simulink model "photovoltaic_single_phase_gridconnected_inverter_5kW"  (R2020b)
settings: Solver=FixedStepDiscrete  StartTime=0.0  StopTime=6  FixedStep=5e-7  MaxStep=1e-6  RelTol=1e-3
undefined symbols (not defined in the file): DiscIntNeverNeededParam, sigbuilder_block
libraries: powerlib x20, pid_lib x2, discretizing x2, re_lib x1, powerlib_meascontrol x1
settings Model: SimulationMode=accelerator  Creator=zhaoy  LastModifiedBy=Administrator
settings DataIOCC: ReturnWorkspaceOutputs=off
settings OptimizationCC: LifeSpan=inf
settings DebuggingCC: ArithmeticOperatorsInVariantConditions=warning
settings SFSimCC: SimUseLocalCustomCode=off  CustomCodeUndefinedFunction=UseInterfaceOnly
settings RTWCC: RTWUseLocalCustomCode=off
settings CodeAppCC: StateflowObjectComments=on
settings SimscapeCC: SimscapeNormalizeSystem=off

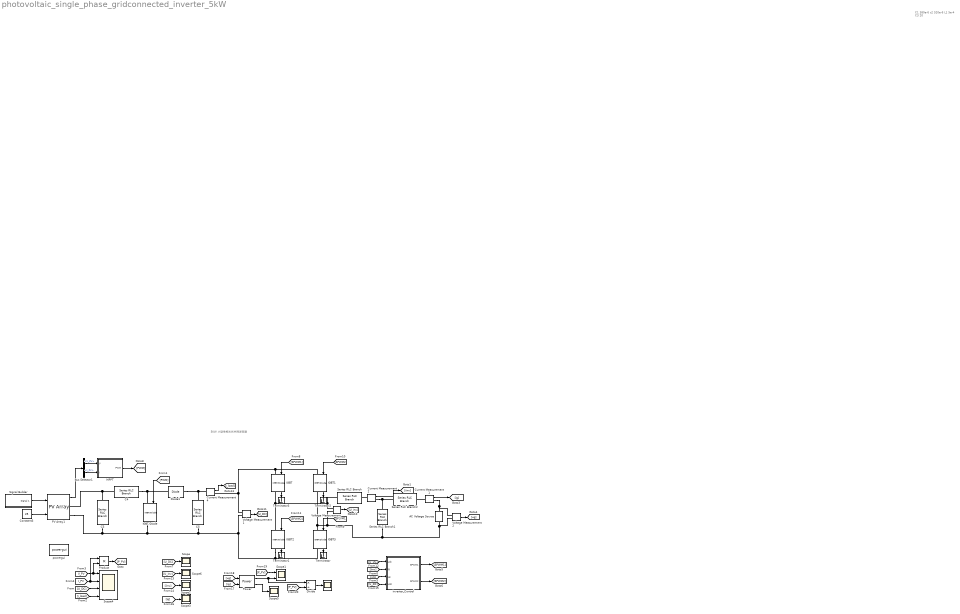
== system photovoltaic_single_phase_gridconnected_inverter_5kW ==
  note: 5KW 小型单相光伏并网逆变器
  note: C1 380e-6
      | c2 520e-6
      | L1 5e-4
      | C3 20
  " " : Scope
  AC Voltage Source : powerlib/Electrical Sources/AC Voltage Source  Amplitude=311  Phase=0  Frequency=50  SampleTime=0  Measurements=None  BusType=swing  Pref=10e3  Qref=0  Qmin=-inf  Qmax=+inf
  Bus Selector1 : BusSelector  OutputSignals=V_PV,I_PV
  C3 : powerlib/Elements/Series RLC Branch  LConnTagsString=__new0  RConnTagsString=__new0  BranchType=C  Resistance=1e-4  Inductance=3.05e-3  SetiL0=off  InitialCurrent=0  Capacitance=500e-6  Setx0=off  InitialVoltage=0  Measurements=Branch voltage
  C4 : powerlib/Elements/Series RLC Branch  LConnTagsString=__new0  RConnTagsString=__new0  BranchType=RL  Resistance=0.01  Inductance=2e-3  SetiL0=off  InitialCurrent=0  Capacitance=100e-6  Setx0=off  InitialVoltage=0  Measurements=Branch voltage
  C5 : powerlib/Elements/Series RLC Branch  LConnTagsString=__new0  RConnTagsString=__new0  BranchType=C  Resistance=1e-4  Inductance=3.05e-3  SetiL0=off  InitialCurrent=0  Capacitance=3000e-6  Setx0=off  InitialVoltage=0  Measurements=Branch voltage
  Constant3 : Constant  Value=25
  Current Measurement1 : powerlib/Measurements/Current Measurement  PhasorSimulation=off  OutputType=Complex  PSBequivalent=0
  Current Measurement2 : powerlib/Measurements/Current Measurement  PhasorSimulation=off  OutputType=Complex  PSBequivalent=0
  Current Measurement4 : powerlib/Measurements/Current Measurement  PhasorSimulation=off  OutputType=Complex  PSBequivalent=0
  Diode1 : powerlib/Power Electronics/Diode  Ron=0.001  Lon=0  Vf=0.8  IC=0  UseSnubber=off  Rs=500  Cs=250e-9  Measurements=off
  Divide : Product  Inputs=*/
  IGBT{,1..3} (4 alike) : powerlib/Power Electronics/IGBT//Diode  Ron=1e-3  Rs=1e5  Cs=inf  Measurements=on
  IGBT/Diode : powerlib/Power Electronics/IGBT//Diode  Ron=1e-3  Rs=1e5  Cs=inf  Measurements=on
  MPPT : Subsystem
  PV Array1 : re_lib/Solar/PV Array  Npar=3  Nser=8  PlotType=array @ 25 deg.C & specified irradiances  S_vec=[600 1000 800]  Temp_C_vec="[ 45 25  ]"  ModuleName=User-defined  PlotWhenSelected=off  Pm=213.15  Ncell=60  Voc=36.3  Isc=7.84  Vm=29  Im=7.35  beta_Voc_pc=-0.36099  alpha_Isc_pc=0.102  beta_Voc=-0.13104  alpha_Isc=0.0079968  IL=7.8654  I0=2.9273e-10  nI=0.98119  Rsh=313.0553  Rs=0.39381  RobustModel=off  RobustCellTemperature=313.3991  BAL=on  Tc=1e-6  Tfilter=5e-5
  Power : powerlib_meascontrol/Measurements/Power  Freq=50  Vinit=[1, 0]  Iinit=[1, 0]  Ts=1e-6
  Product : Product
  Scope{,2..3,5..6} (5 alike) : Scope
  Scope1 : Scope  NumInputPorts=2
  Scope4 : Scope  NumInputPorts=4
  Series RLC Branch : powerlib/Elements/Series RLC Branch  LConnTagsString=__new0  RConnTagsString=__new0  BranchType=L  Resistance=0.01  Inductance=4.06e-3  SetiL0=off  InitialCurrent=0  Capacitance=1e-6  Setx0=off  InitialVoltage=0  Measurements=None
  Series RLC Branch1 : powerlib/Elements/Series RLC Branch  LConnTagsString=__new0  RConnTagsString=__new0  BranchType=C  Resistance=0.01  Inductance=20e-3  SetiL0=off  InitialCurrent=0  Capacitance=6.23e-6  Setx0=off  InitialVoltage=0  Measurements=None
  Series RLC Branch2 : powerlib/Elements/Series RLC Branch  LConnTagsString=__new0  RConnTagsString=__new0  BranchType=L  Resistance=0.01  Inductance=4.35e-3  SetiL0=off  InitialCurrent=0  Capacitance=1e-6  Setx0=off  InitialVoltage=0  Measurements=None
  Signal Builder : Subsystem  Tag=STV Subsys  LoadFcn=sigbuilder_block('load');  StartFcn=sigbuilder_block('start');  StopFcn=sigbuilder_block('stop');  ClipboardFcn=sigbuilder_block('clipboard');  mask(Sigbuilder block){tuvar=[0:10]}
      mask help: Simulink:masks:SigbuilderBlock_MD
      mask init:
      | if ~strcmp(get_param(bdroot(gcbh),'SimulationStatus'),'stopped') tuvar = sigbuilder_block('maskInit'); end
      settings: CopyFcn=sigbuilder_block('copy');  DeleteFcn=sigbuilder_block('delete');  ModelCloseFcn=sigbuilder_block('modelClose');  PreSaveFcn=sigbuilder_block('preSave');  PauseFcn=sigbuilder_block('pause');  ContinueFcn=sigbuilder_block('continue');  NameChangeFcn=sigbuilder_block('namechange');  OpenFcn=sigbuilder_block('open',[437.6 199.2 550.4 400 ]);  CloseFcn=sigbuilder_block('close');
      mask Display: plot(0, 0, 100, 100,[2, 2, 32, 32, 2], [68, 8, 8, 68, 68],[32, 2], [38, 38], [32, 19, 2],[53, 60, 44], [32, 17, 17, 2],[16, 16, 31, 31]);txt = getActiveGroup(gcbh);text(2, 100, txt,'verticalAlignment', 'top');
  Terminator{,1..3} (4 alike) : Terminator
  Voltage Measurement1 : powerlib/Measurements/Voltage Measurement  PhasorSimulation=off  OutputType=Complex  PSBequivalent=0
  Voltage Measurement2 : powerlib/Measurements/Voltage Measurement  PhasorSimulation=off  OutputType=Complex  PSBequivalent=0
  Voltage Measurement3 : powerlib/Measurements/Voltage Measurement  PhasorSimulation=off  OutputType=Complex  PSBequivalent=0
  inverter_Control : Subsystem
  powergui : powerlib/powergui  Priority=1  SimulationMode=Discrete  SampleTime=1e-6  frequency=50  Iterations=50  frequencyindice=50  Pbase=100e6  ErrMax=1e-4  UnitsV=kV  UnitsW=MW  buscounter=0  FunctionMessages=off  echomessages=off  EnableUseOfTLC=off  CurrentSourceSwitches=off  DisableSnubberDevices=off  DisableRonSwitches=off  DisableVfSwitches=off  DisplayEquations=off  AutomaticDiscreteSolvers=off  SolverType=Tustin/Backward Euler (TBE)  Interpol=off  ExternalGateDelay=off  methode=off  Ts=10  x0status=blocks  SPID=off  SwTol=0  HookPort=off  NonlinearTolerance=1e-4  nMaxIteration=100  ContinueOnMaxIteration=off  RestoreLinks=warning  ResistiveCurrentMeasurement=off  Frange=[0:2:500]  Ylog=off  Xlog=on  ShowGrid=off  save=off  variable=ZData  structure=ScopeData2  ZoomFFT=off  StartTime=1  cycles=40  DisplayStyle=2  fundamental=50  FreqAxis=on  MaxFrequency=1000  frequencyindicesteady=1  RmsSteady=2  display=off
  wires:
  Constant3/1 -> PV Array1/2
  Signal Builder/1(Signal 1) -> PV Array1/1
  PV Array1/1 -> Bus Selector1/1
  Voltage Measurement1/1 -> [U_DC]
  Current Measurement4/1 -> [i_load]
  [U_DC] -> Scope4/3
  [i_load] -> Scope4/4
  [V_PV] -> Product/2, Scope4/1
  [I_PV] -> Product/1, Scope4/2
  Current Measurement1/1 -> [ig]
  [SPWM1] -> IGBT/1
  [SPWM2] -> IGBT1/1
  Voltage Measurement2/1 -> [ug]
  [SPWM1] -> IGBT3/1
  [SPWM2] -> IGBT2/1
  inverter_Control/2(SPWM2) -> [SPWM2]
  [U_DC] -> inverter_Control/1(udc)
  [iinv] -> inverter_Control/2(Ig)
  inverter_Control/1(SPWM1) -> [SPWM1]
  Current Measurement2/1 -> [iinv]
  [ug] -> inverter_Control/3(ug)
  [U_DC] -> inverter_Control/4(Udc)
  Voltage Measurement3/1 -> [U_inv]
  [PWM] -> IGBT/Diode/1
  Bus Selector1/1 -> MPPT/1(V)  "<V_PV>"
  Bus Selector1/2 -> MPPT/2(I)  "<I_PV>"
  IGBT3/1 -> Terminator/1
  IGBT2/1 -> Terminator1/1
  IGBT1/1 -> Terminator2/1
  IGBT/1 -> Terminator3/1
  MPPT/1(PWM) -> [PWM]
  [U_DC] -> Scope/1
  [U_inv] -> Scope6/1
  [iinv] -> Scope2/1
  [ig] -> Scope3/1
  Product/1 -> [P_PV]
  [ig] -> Power/2
  [ug] -> Power/1
  Power/2 -> Scope5/1
  [P_PV] -> Scope1/1
  Power/1 -> Divide/1, Scope1/2
  Divide/1 -> " "/1
  [P_PV] -> Divide/2
  connections:
  IGBT3/RConn1 -- PV Array1/RConn2 -- C3/RConn1 -- IGBT/Diode/RConn1 -- C5/RConn1 -- Voltage Measurement1/LConn2 -- IGBT2/RConn1
  Current Measurement4/LConn1 -- Diode1/RConn1 -- C5/LConn1
  IGBT/LConn1 -- Voltage Measurement1/LConn1 -- Current Measurement4/RConn1 -- IGBT1/LConn1
  Voltage Measurement2/LConn1 -- Current Measurement1/RConn1 -- AC Voltage Source/RConn1
  Voltage Measurement2/LConn2 -- Series RLC Branch1/RConn1 -- Voltage Measurement3/LConn2 -- IGBT1/RConn1 -- IGBT3/LConn1 -- AC Voltage Source/LConn1
  Series RLC Branch/LConn1 -- Voltage Measurement3/LConn1 -- IGBT/RConn1 -- IGBT2/LConn1
  Current Measurement2/LConn1 -- Series RLC Branch/RConn1
  Current Measurement2/RConn1 -- Series RLC Branch2/LConn1 -- Series RLC Branch1/LConn1
  Current Measurement1/LConn1 -- Series RLC Branch2/RConn1
  C3/LConn1 -- C4/LConn1 -- PV Array1/RConn1
  C4/RConn1 -- Diode1/LConn1 -- IGBT/Diode/LConn1

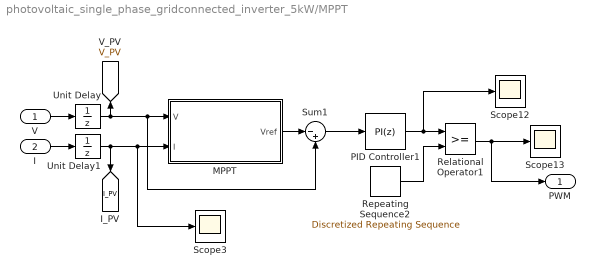
== system photovoltaic_single_phase_gridconnected_inverter_5kW/MPPT ==
  V : Inport
  I : Inport  Port=2
  MPPT : MATLAB Function  TreatAsAtomicUnit=on
  PID Controller1 : pid_lib/PID Controller  Controller=PI  Form=Parallel  TimeDomain=Discrete-time  UseExternalTs=off  SampleTime=-1  IntegratorMethod=Forward Euler  FilterMethod=Forward Euler  ControllerParametersSource=internal  P=0.005  I=0.0075  D=0  UseFilter=on  N=100  TunerSelectOption=Transfer Function Based (PID Tuner App)  InitialConditionSource=internal  InitialConditionForIntegrator=0  InitialConditionForFilter=0  DifferentiatorICPrevScaledInput=0  ExternalReset=none  TrackingMode=off  Kt=1  LimitOutput=off  SatLimitsSource=internal  UpperSaturationLimit=inf  LowerSaturationLimit=-inf  LinearizeAsGain=on  AntiWindupMode=none  Kb=1  POutMin=[]  POutMax=[]  IOutMin=[]  IOutMax=[]  DOutMin=[]  DOutMax=[]  NOutMin=[]  NOutMax=[]  SumOutMin=[]  SumOutMax=[]  SaturationOutMin=[]  SaturationOutMax=[]  PParamMin=[]  PParamMax=[]  IParamMin=[]  IParamMax=[]  DParamMin=[]  DParamMax=[]  NParamMin=[]  NParamMax=[]  KbParamMin=[]  KbParamMax=[]  KtParamMin=[]  KtParamMax=[]  KbOutMin=[]  KbOutMax=[]  KtOutMin=[]  KtOutMax=[]  IntegratorOutMin=[]  IntegratorOutMax=[]  FilterOutMin=[]  FilterOutMax=[]  SumI1OutMin=[]  SumI1OutMax=[]  SumI2OutMin=[]  SumI2OutMax=[]  SumI3OutMin=[]  SumI3OutMax=[]  SumI4OutMin=[]  SumI4OutMax=[]  SumDOutMin=[]  SumDOutMax=[]  DifferentiatorOutMin=[]  DifferentiatorOutMax=[]  FilterDiffOutCoefMin=[]  FilterDiffOutCoefMax=[]  ReciprocalOutMin=[]  ReciprocalOutMax=[]  SumDenOutMin=[]  SumDenOutMax=[]  SumNumOutMin=[]  SumNumOutMax=[]  DivideOutMin=[]  DivideOutMax=[]  UdiffTsProdOutMin=[]  UdiffTsProdOutMax=[]  NTsProdOutMin=[]  NTsProdOutMax=[]  UintegralTsProdOutMin=[]  UintegralTsProdOutMax=[]  UngainTsProdOutMin=[]  UngainTsProdOutMax=[]  IntegratorContinuousStateAttributes=''  IntegratorStateMustResolveToSignalObject=off  IntegratorRTWStateStorageClass=Auto  FilterContinuousStateAttributes=''  FilterStateMustResolveToSignalObject=off  FilterRTWStateStorageClass=Auto  ParallelPVariant=InternalParameters  IdealPVariant=Disabled  IVariant=InternalParameters  DVariant=Disabled  IntegratorVariant=Discrete  SatVariant=Disabled  AWVariant=Passthrough  PCopyVariant=Disabled  TRVariant=Disabled  FdbkBlocksVariant=Forward  IdealPFdbkVariant=Disabled  SatFdbkVariant=Disabled  DerivativeFilterVariant=Disabled  NVariant=Disabled  NCopyVariant=Disabled_SignalSpec  FilterICVariant=Disabled  IntegratorICVariant=InternalICs  ExternalResetVariant=Disabled  TRSumVariant=Passthrough  SumFdbkVariant=Disabled  SumVariant=Sum_PI  TsampFilterVariant=InternalTs  TsampNgainVariant=Passthrough  TsampIntegralVariant=Passthrough  ExternalSaturationOutDataTypeStr=Inherit: Same as second input
  Relational Operator1 : RelationalOperator  OutDataTypeStr=boolean  RndMeth=Simplest
  Repeating Sequence2 : discretizing/Discretized Repeating Sequence  rep_seq_t=[0 0.0001 0.0002]  rep_seq_y=[0 1 0]  SampleTime=1e-6
      settings: SourceProductBaseCode=SL
  Scope12 : Scope
  Scope13 : Scope
  Scope3 : Scope
  Sum1 : Sum  Inputs=|-+
  Unit Delay : UnitDelay  SampleTime=1e-5  HasFrameUpgradeWarning=on
  Unit Delay1 : UnitDelay  SampleTime=1e-5  HasFrameUpgradeWarning=on
  PWM : Outport
  tag scope: I_PV=global, V_PV=global
  wires:
  Relational Operator1/1 -> PWM/1, Scope13/1
  Unit Delay1/1 -> [I_PV], MPPT/2(I), Scope3/1
  MPPT/1(Vref) -> Sum1/1
  PID Controller1/1 -> Scope12/1, Relational Operator1/1
  Repeating Sequence2/1 -> Relational Operator1/2
  Sum1/1 -> PID Controller1/1
  V/1 -> Unit Delay/1
  I/1 -> Unit Delay1/1
  Unit Delay/1 -> [V_PV], MPPT/1(V), Sum1/2

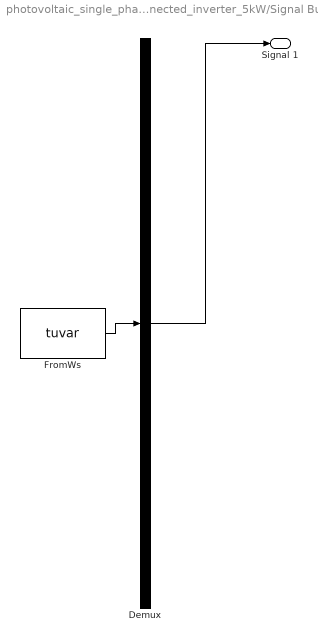
== system photovoltaic_single_phase_gridconnected_inverter_5kW/Signal Builder ==
  Demux : Demux  Tag=STV Demux  Outputs=1
      settings: DisplayOption=none
  FromWs : FromWorkspace  Tag=STV FromWs  VariableName=tuvar
      SigBuilderData=|
      | common.afterFinalStr = 'Extrapolate'
      | common.sampleTime = 0
      | dataSet.timeRange = [0 10]
      | dataSet.name = 'Group 1'
      | sbobj.Groups.Name = 'Group 1'
      | sbobj.Groups.Signals.Name = 'Signal 1'
      | sbobj.Groups.Signals.XData = [0 2 2 4 4 6 10]
      | sbobj.Groups.Signals.YData = [600 600 1000 1000 800 800 800]
  Signal 1 : Outport  Tag=STV Outport
  wires:
  Demux/1 -> Signal 1/1
  FromWs/1 -> Demux/1

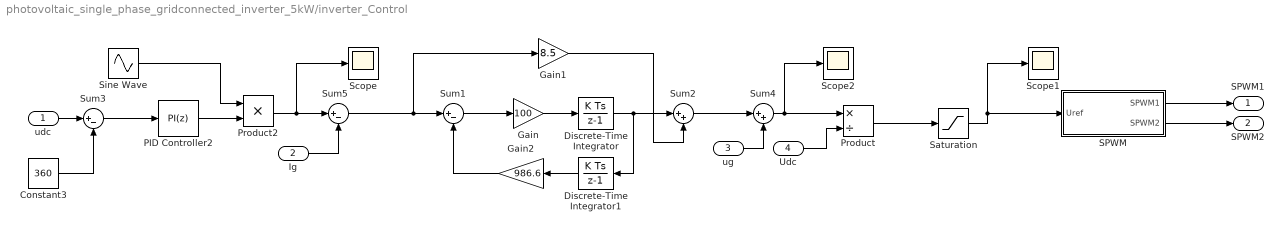
== system photovoltaic_single_phase_gridconnected_inverter_5kW/inverter_Control ==
  udc : Inport
  Ig : Inport  Port=2
  ug : Inport  Port=3
  Udc : Inport  Port=4
  Constant3 : Constant  Value=360
  Discrete-Time Integrator : DiscreteIntegrator  SampleTime=-1  ICPrevOutput=DiscIntNeverNeededParam  ICPrevScaledInput=DiscIntNeverNeededParam
  Discrete-Time Integrator1 : DiscreteIntegrator  SampleTime=-1  ICPrevOutput=DiscIntNeverNeededParam  ICPrevScaledInput=DiscIntNeverNeededParam
  Gain : Gain  Gain=100
  Gain1 : Gain  Gain=8.5
  Gain2 : Gain  Gain=986.6
  PID Controller2 : pid_lib/PID Controller  Controller=PI  Form=Parallel  TimeDomain=Discrete-time  UseExternalTs=off  SampleTime=-1  IntegratorMethod=Forward Euler  FilterMethod=Forward Euler  ControllerParametersSource=internal  P=0.6  I=10  D=0  UseFilter=on  N=100  TunerSelectOption=Transfer Function Based (PID Tuner App)  InitialConditionSource=internal  InitialConditionForIntegrator=0  InitialConditionForFilter=0  DifferentiatorICPrevScaledInput=0  ExternalReset=none  TrackingMode=off  Kt=1  LimitOutput=off  SatLimitsSource=internal  UpperSaturationLimit=1  LowerSaturationLimit=-1  LinearizeAsGain=on  AntiWindupMode=none  Kb=1  POutMin=[]  POutMax=[]  IOutMin=[]  IOutMax=[]  DOutMin=[]  DOutMax=[]  NOutMin=[]  NOutMax=[]  SumOutMin=[]  SumOutMax=[]  SaturationOutMin=[]  SaturationOutMax=[]  PParamMin=[]  PParamMax=[]  IParamMin=[]  IParamMax=[]  DParamMin=[]  DParamMax=[]  NParamMin=[]  NParamMax=[]  KbParamMin=[]  KbParamMax=[]  KtParamMin=[]  KtParamMax=[]  KbOutMin=[]  KbOutMax=[]  KtOutMin=[]  KtOutMax=[]  IntegratorOutMin=[]  IntegratorOutMax=[]  FilterOutMin=[]  FilterOutMax=[]  SumI1OutMin=[]  SumI1OutMax=[]  SumI2OutMin=[]  SumI2OutMax=[]  SumI3OutMin=[]  SumI3OutMax=[]  SumI4OutMin=[]  SumI4OutMax=[]  SumDOutMin=[]  SumDOutMax=[]  DifferentiatorOutMin=[]  DifferentiatorOutMax=[]  FilterDiffOutCoefMin=[]  FilterDiffOutCoefMax=[]  ReciprocalOutMin=[]  ReciprocalOutMax=[]  SumDenOutMin=[]  SumDenOutMax=[]  SumNumOutMin=[]  SumNumOutMax=[]  DivideOutMin=[]  DivideOutMax=[]  UdiffTsProdOutMin=[]  UdiffTsProdOutMax=[]  NTsProdOutMin=[]  NTsProdOutMax=[]  UintegralTsProdOutMin=[]  UintegralTsProdOutMax=[]  UngainTsProdOutMin=[]  UngainTsProdOutMax=[]  IntegratorContinuousStateAttributes=''  IntegratorStateMustResolveToSignalObject=off  IntegratorRTWStateStorageClass=Auto  FilterContinuousStateAttributes=''  FilterStateMustResolveToSignalObject=off  FilterRTWStateStorageClass=Auto  ParallelPVariant=InternalParameters  IdealPVariant=Disabled  IVariant=InternalParameters  DVariant=Disabled  IntegratorVariant=Discrete  SatVariant=Disabled  AWVariant=Passthrough  PCopyVariant=Disabled  TRVariant=Disabled  FdbkBlocksVariant=Forward  IdealPFdbkVariant=Disabled  SatFdbkVariant=Disabled  DerivativeFilterVariant=Disabled  NVariant=Disabled  NCopyVariant=Disabled_SignalSpec  FilterICVariant=Disabled  IntegratorICVariant=InternalICs  ExternalResetVariant=Disabled  TRSumVariant=Passthrough  SumFdbkVariant=Disabled  SumVariant=Sum_PI  TsampFilterVariant=InternalTs  TsampNgainVariant=Passthrough  TsampIntegralVariant=Passthrough  ExternalSaturationOutDataTypeStr=Inherit: Same as second input
  Product : Product  Inputs=*/
  Product2 : Product
  SPWM : Subsystem
  Saturation : Saturate  UpperLimit=1  LowerLimit=-1
  Scope : Scope
  Scope1 : Scope
  Scope2 : Scope
  Sine Wave : Sin  Frequency=100*pi  SampleTime=0
  Sum1 : Sum  Inputs=|+-
  Sum2 : Sum  Inputs=|++
  Sum3 : Sum  Inputs=|+-
  Sum4 : Sum  Inputs=|++
  Sum5 : Sum  Inputs=|+-
  SPWM1 : Outport
  SPWM2 : Outport  Port=2
  wires:
  Constant3/1 -> Sum3/2
  Sum3/1 -> PID Controller2/1
  udc/1 -> Sum3/1
  PID Controller2/1 -> Product2/2
  Sine Wave/1 -> Product2/1
  Ig/1 -> Sum5/2
  Saturation/1 -> SPWM/1(Uref), Scope1/1
  Product2/1 -> Scope/1, Sum5/1
  Sum2/1 -> Sum4/1
  ug/1 -> Sum4/2
  Sum4/1 -> Scope2/1, Product/1
  Udc/1 -> Product/2
  Product/1 -> Saturation/1
  SPWM/1(SPWM1) -> SPWM1/1
  SPWM/2(SPWM2) -> SPWM2/1
  Sum5/1 -> Gain1/1, Sum1/1
  Discrete-Time Integrator1/1 -> Gain2/1
  Gain/1 -> Discrete-Time Integrator/1
  Sum1/1 -> Gain/1
  Gain1/1 -> Sum2/2
  Gain2/1 -> Sum1/2
  Discrete-Time Integrator/1 -> Discrete-Time Integrator1/1, Sum2/1

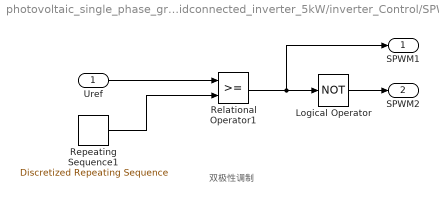
== system photovoltaic_single_phase_gridconnected_inverter_5kW/inverter_Control/SPWM ==
  note: 双极性调制
  Uref : Inport
  Logical Operator : Logic  Operator=NOT  AllPortsSameDT=off  OutDataTypeStr=boolean
  Relational Operator1 : RelationalOperator  OutDataTypeStr=boolean  RndMeth=Simplest
  Repeating Sequence1 : discretizing/Discretized Repeating Sequence  rep_seq_t=[0 0.00005 0.0001]  rep_seq_y=[-1 1 -1]  SampleTime=1e-6
      settings: SourceProductBaseCode=SL
  SPWM1 : Outport
  SPWM2 : Outport  Port=2
  wires:
  Uref/1 -> Relational Operator1/1
  Logical Operator/1 -> SPWM2/1
  Repeating Sequence1/1 -> Relational Operator1/2
  Relational Operator1/1 -> SPWM1/1, Logical Operator/1

== matlab function photovoltaic_single_phase_gridconnected_inverter_5kW/MPPT/MPPT ==
  data: V input; Vref output; I input
function Vref = MPPT_algorithm_V(V,I)
Vrefmax = 300;
Vrefmin = 0;
Vrefinit = 200;
deltaVref = 0.002;
persistent Vold Pold Vrefold;
dataType = 'double';
if isempty(Vold)
    Vold = 0;
    Pold = 0;
    Vrefold = Vrefinit;
end
P = V*I;
dV = V - Vold;
dP = P - Pold;

if dP~= 0
    if dP<0
        if dV<0
            Vref = Vrefold + deltaVref;
        else
            Vref = Vrefold - deltaVref;
        end
    else
         if dV<0
            Vref = Vrefold - deltaVref;
        else
            Vref = Vrefold + deltaVref;
         end
    end
else
    Vref = Vrefold;
end
if Vref >= Vrefmax || Vref <=Vrefmin
    Vref = Vrefold;
end
Vrefold = Vref;
Vold = V;
Pold = P;
